simulink model "discrete_controller"  (R2021b)
settings: Solver=VariableStepAuto  StartTime=0.0  StopTime=60*60*24*60  RelTol=1e-3
values from neighbouring files (symbols this model uses):
  alpha = 3.7541    [Parameters.m]
  beta = beta/(24*60*60)    (= 1.57476851852e-05)    [Parameters.m]
  dI = dI/(24*60*60)    (= 1.15740740741e-06)    [Parameters.m]
  dV = dV/(24*60*60)    (= 2.13148148148e-05)    [Parameters.m]
  I0 = 0    [Parameters.m]
  Kf_d = place(A1_d,B1_d,p0_d)    [control_design.m]
  L = 936.4293    [Parameters.m]
  r = r/(24*60*60)    (= 6.97916666667e-07)    [Parameters.m]
  S0 = 128.1481    [Parameters.m]
  Ts = 2*86400    (= 172800)    [control_design.m]
  V0 = 0    [Parameters.m]
settings Model: Creator=chenx  LastModifiedBy=chenx

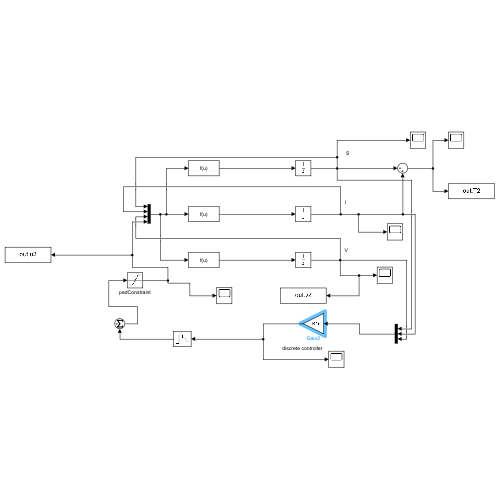
[thumbnail: Simulink's stored preview of the top-level diagram]
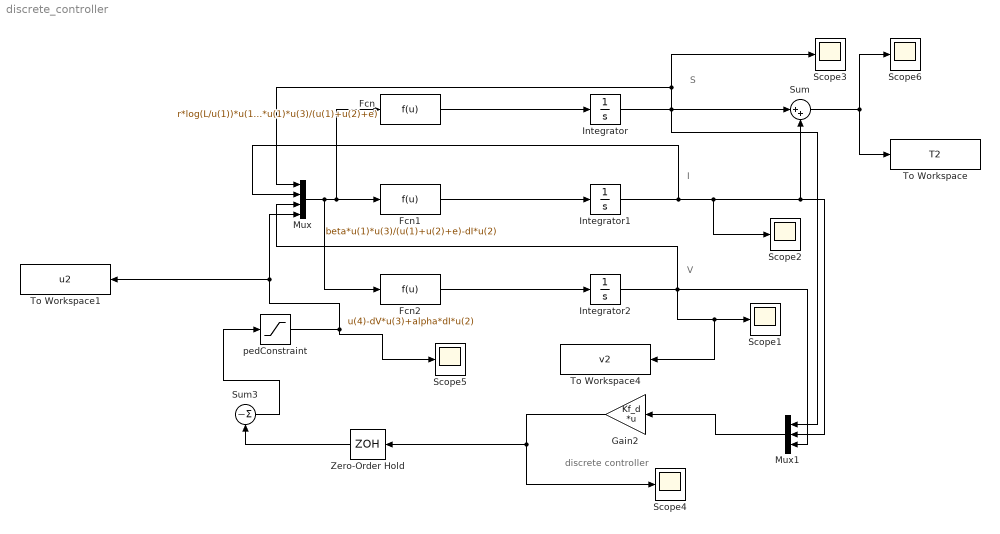
== system discrete_controller ==
  note: discrete controller
  note: V
  note: I
  note: S
  Fcn : Fcn  Expr=r*log(L/u(1))*u(1)-beta*u(1)*u(3)/(u(1)+u(2)+e)
  Fcn1 : Fcn  Expr=beta*u(1)*u(3)/(u(1)+u(2)+e)-dI*u(2)
  Fcn2 : Fcn  Expr=u(4)-dV*u(3)+alpha*dI*u(2)
  Gain2 : Gain  Gain=Kf_d  Multiplication=Matrix(K*u)
  Integrator : Integrator  InitialCondition=S0
  Integrator1 : Integrator  InitialCondition=I0
  Integrator2 : Integrator  InitialCondition=V0
  Mux : Mux
  Mux1 : Mux  Inputs=3
  Scope{1..6} (6 alike) : Scope
  Sum : Sum  Inputs=|++
  Sum3 : Sum  Inputs=|-
  To Workspace : ToWorkspace  VariableName=T2  SampleTime=-1
  To Workspace1 : ToWorkspace  VariableName=u2  SaveFormat=Timeseries  SampleTime=-1
  To Workspace4 : ToWorkspace  VariableName=v2  SampleTime=-1
  Zero-Order Hold : ZeroOrderHold  SampleTime=Ts
  pedConstraint : Saturate  UpperLimit=1000  LowerLimit=0
  wires:
  Integrator2/1 -> To Workspace4/1, Scope1/1, Mux1/3, Mux/3
  Mux1/1 -> Gain2/1
  Fcn1/1 -> Integrator1/1
  Mux/1 -> Fcn2/1, Fcn1/1, Fcn/1
  Sum/1 -> To Workspace/1, Scope6/1
  Integrator/1 -> Scope3/1, Mux/1, Mux1/1, Sum/1
  Integrator1/1 -> Mux1/2, Sum/2, Scope2/1, Mux/2
  Fcn/1 -> Integrator/1
  Fcn2/1 -> Integrator2/1
  Gain2/1 -> Zero-Order Hold/1, Scope4/1
  Zero-Order Hold/1 -> Sum3/1
  Sum3/1 -> pedConstraint/1
  pedConstraint/1 -> Scope5/1, Mux/4, To Workspace1/1
